simulink model "Simulationes"  (R2024a)
settings: Solver=VariableStepAuto  StartTime=0.0  StopTime=20  RelTol=1e-3
undefined symbols (not defined in the file): Ad, Bd, Cd, Dd, Discrete, Input_Step, K_discrete, Time
libraries: simulink x1, ctrlSharedLib x1
settings Model: Creator=eduar  LastModifiedBy=eduar

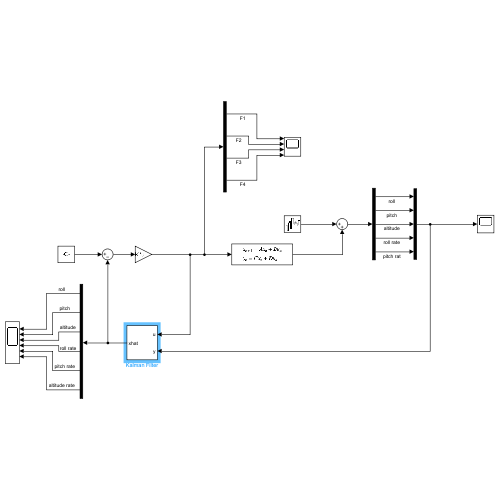
[thumbnail: Simulink's stored preview of the top-level diagram]
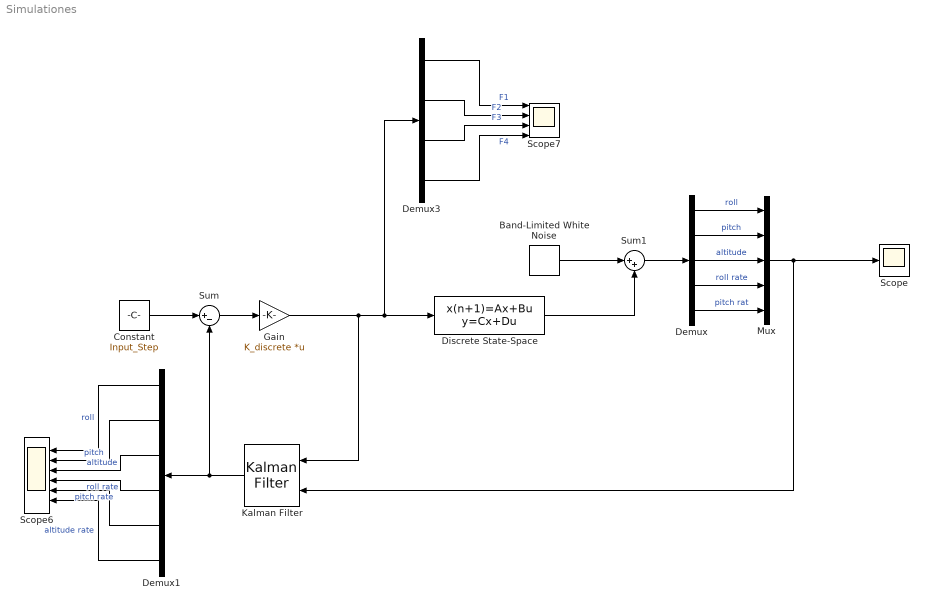
== system Simulationes ==
  Band-Limited White Noise : simulink/Sources/Band-Limited White Noise  Cov=[0.00005]  Ts=0.02  seed=[2331]
  Constant : Constant  Value=Input_Step
  Demux : Demux  Outputs=5
  Demux1 : Demux  Outputs=6
  Demux3 : Demux
  Discrete State-Space : DiscreteStateSpace  A=Ad  B=Bd  C=Cd  D=Dd  SampleTime=0.02
  Gain : Gain  Gain=K_discrete  Multiplication=Matrix(K*u)
  Kalman Filter : ctrlSharedLib/Kalman Filter  TimeDomain=Discrete-Time  UseCurrentEstimator=on  ModelSource=Individual A, B, C, D matrices  ModelSourceVariable=ss(0.95,1,1,0,1)  A=Ad  B=Bd  C=Cd  D=Dd  NumberOfStates=1  NumberOfInputs=1  NumberOfOutputs=1  InitialEstimateSource=Dialog  X0=0  P0=10  UseK=off  UseGH=off  NumberOfProcessNoiseInputs=1  G=1  TimeInvariantG=on  H=0  TimeInvariantH=on  Q=diag([0,0,0,0.0000001,0.0000001,0.0000001])  TimeInvariantQ=on  R=1  TimeInvariantR=on  N=0  TimeInvariantN=on  AddInputPort=on  AddEnablePort=off  OutputEstimatedY=off  OutputP=off  Ts=0.02
  Mux : Mux  Inputs=5
  Scope : Scope
  Scope6 : Scope  NumInputPorts=6
  Scope7 : Scope  NumInputPorts=4
  Sum : Sum  Inputs=|+-
  Sum1 : Sum  Inputs=|++
  wires:
  Constant/1 -> Sum/1
  Sum/1 -> Gain/1
  Gain/1 -> Kalman Filter/1, Demux3/1, Discrete State-Space/1
  Kalman Filter/1 -> Sum/2, Demux1/1
  Band-Limited White Noise/1 -> Sum1/1
  Sum1/1 -> Demux/1
  Demux/1 -> Mux/1  "roll"
  Demux/2 -> Mux/2  "pitch"
  Demux/3 -> Mux/3  "altitude"
  Demux/4 -> Mux/4  "roll rate"
  Demux/5 -> Mux/5  "pitch rat"
  Mux/1 -> Scope/1, Kalman Filter/2
  Discrete State-Space/1 -> Sum1/2
  Demux1/1 -> Scope6/1  "roll"
  Demux1/2 -> Scope6/2  "pitch"
  Demux1/3 -> Scope6/3  "altitude"
  Demux1/4 -> Scope6/4  "roll rate"
  Demux1/5 -> Scope6/5  "pitch rate"
  Demux1/6 -> Scope6/6  "altitude rate"
  Demux3/1 -> Scope7/1  "F1"
  Demux3/2 -> Scope7/2  "F2"
  Demux3/3 -> Scope7/3  "F3"
  Demux3/4 -> Scope7/4  "F4"
